simulink model "csu_tdl_thruster_dynamics_lander_hrn"  (R2014b)
settings: Solver=FixedStepDiscrete  StartTime=t0  StopTime=tFinal  FixedStep=sim_dt  RelTol=1e-3
libraries: csu_tdl_thruster_dynamics_lander_lib x1
settings Model: Creator=escrane  LastModifiedBy=mstewart
settings DebuggingCC: UnderspecifiedInitializationDetection=Classic  MergeDetectMultiDrivingBlocksExec=none

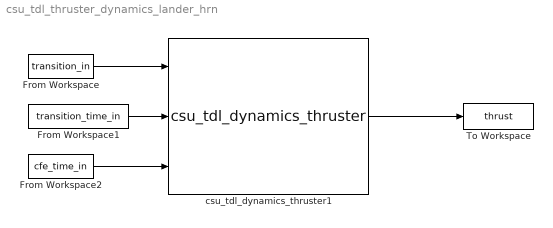
== system csu_tdl_thruster_dynamics_lander_hrn ==
  From Workspace : FromWorkspace  VariableName=transition_in  SampleTime=0
  From Workspace1 : FromWorkspace  VariableName=transition_time_in  SampleTime=0
  From Workspace2 : FromWorkspace  VariableName=cfe_time_in  SampleTime=0
  To Workspace : ToWorkspace  VariableName=thrust  SaveFormat=Timeseries  SampleTime=-1
  csu_tdl_dynamics_thruster1 : csu_tdl_thruster_dynamics_lander_lib/csu_tdl_dynamics_thruster  thruster_idx=test_thruster_id  time_since_rise_lookup=tdl_thruster1_rising_lookup_time  thrust_rising_output_lookup=tdl_thruster1_rising_lookup_thrust  time_since_fall_lookup=tdl_thruster1_falling_lookup_time  thrust_falling_output_lookup=tdl_thruster1_falling_lookup_thrust  thrust_noise_mean=tdl_thruster1_thrust_noise_mean  thrust_noise_std=tdl_thruster1_thrust_noise_std  thrust_noise_seed=tdl_thruster1_thrust_noise_seed  thrust_noise_on=0
  wires:
  csu_tdl_dynamics_thruster1/1 -> To Workspace/1
  From Workspace/1 -> csu_tdl_dynamics_thruster1/1
  From Workspace1/1 -> csu_tdl_dynamics_thruster1/2
  From Workspace2/1 -> csu_tdl_dynamics_thruster1/3
